simulink model "Slding control"  (R2020b)
settings: Solver=VariableStepAuto  StartTime=0.0  StopTime=50.0  RelTol=1e-3
values from neighbouring files (symbols this model uses):
  A = [-0.0239 -0.0494 0 -32.2 ... (first row only)    [P46091204.m]    (also in Sliding control.m)
  B = [0 ... (first row only)    [P46091204.m]    (also in Sliding control.m = [0 5.05*10^(-5))
  C = eye(4)    [P46091204.m]    (also in Sliding control.m = [K,eye(2)]*T)
  D = [0]    [P46091204.m]    (also in Sliding control.m = -C*A)
settings Model: Creator=ab458  LastModifiedBy=chengying
settings SolverCC: ZeroCrossAlgorithm=Adaptive
settings DebuggingCC: IgnoredZcDiagnostic=none
settings SFSimCC: CustomCodeUndefinedFunction=UseInterfaceOnly

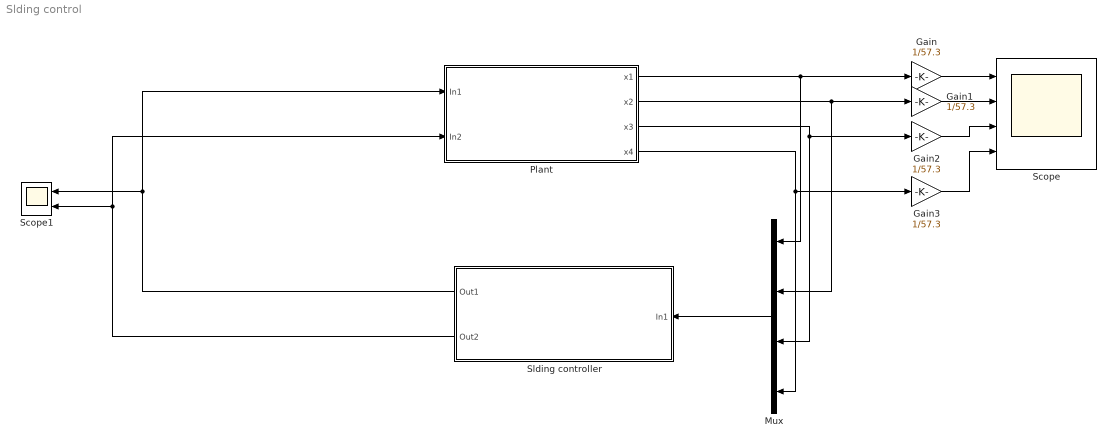
== system Slding control ==
  Gain{,1..3} (4 alike) : Gain  Gain=1/57.3
  Mux : Mux
  Plant : Subsystem
  Scope : Scope  NumInputPorts=4
  Scope1 : Scope  NumInputPorts=2
  Slding controller : Subsystem
  wires:
  Plant/1(x1) -> Mux/1, Gain/1
  Plant/2(x2) -> Mux/2, Gain1/1
  Plant/3(x3) -> Gain2/1, Mux/3
  Plant/4(x4) -> Gain3/1, Mux/4
  Slding controller/1(Out1) -> Plant/1(In1), Scope1/1
  Slding controller/2(Out2) -> Plant/2(In2), Scope1/2
  Mux/1 -> Slding controller/1(In1)
  Gain/1 -> Scope/1
  Gain1/1 -> Scope/2
  Gain2/1 -> Scope/3
  Gain3/1 -> Scope/4

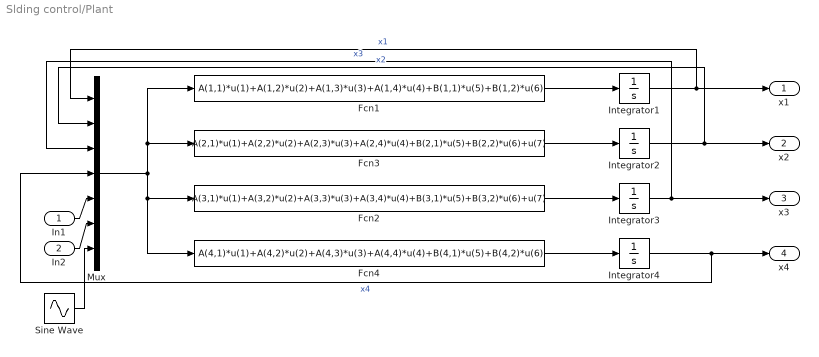
== system Slding control/Plant ==
  In1 : Inport
  In2 : Inport  Port=2
  Fcn1 : Fcn  Expr=A(1,1)*u(1)+A(1,2)*u(2)+A(1,3)*u(3)+A(1,4)*u(4)+B(1,1)*u(5)+B(1,2)*u(6)
  Fcn2 : Fcn  Expr=A(3,1)*u(1)+A(3,2)*u(2)+A(3,3)*u(3)+A(3,4)*u(4)+B(3,1)*u(5)+B(3,2)*u(6)+u(7)
  Fcn3 : Fcn  Expr=A(2,1)*u(1)+A(2,2)*u(2)+A(2,3)*u(3)+A(2,4)*u(4)+B(2,1)*u(5)+B(2,2)*u(6)+u(7)
  Fcn4 : Fcn  Expr=A(4,1)*u(1)+A(4,2)*u(2)+A(4,3)*u(3)+A(4,4)*u(4)+B(4,1)*u(5)+B(4,2)*u(6)
  Integrator1 : Integrator  InitialCondition=1
  Integrator2 : Integrator
  Integrator3 : Integrator  InitialCondition=1
  Integrator4 : Integrator
  Mux : Mux  Inputs=7
  Sine Wave : Sin  Amplitude=0.4  SampleTime=0
  x1 : Outport  VectorParamsAs1DForOutWhenUnconnected=off
  x2 : Outport  Port=2  VectorParamsAs1DForOutWhenUnconnected=off
  x3 : Outport  Port=3  VectorParamsAs1DForOutWhenUnconnected=off
  x4 : Outport  Port=4  VectorParamsAs1DForOutWhenUnconnected=off
  wires:
  Mux/1 -> Fcn3/1, Fcn1/1, Fcn4/1, Fcn2/1
  In2/1 -> Mux/6
  In1/1 -> Mux/5
  Fcn2/1 -> Integrator3/1
  Integrator1/1 -> x1/1, Mux/1  "x1"
  Integrator2/1 -> x2/1, Mux/2  "x2"
  Integrator4/1 -> x4/1, Mux/4  "x4"
  Fcn1/1 -> Integrator1/1
  Fcn4/1 -> Integrator4/1
  Integrator3/1 -> x3/1, Mux/3  "x3"
  Fcn3/1 -> Integrator2/1
  Sine Wave/1 -> Mux/7

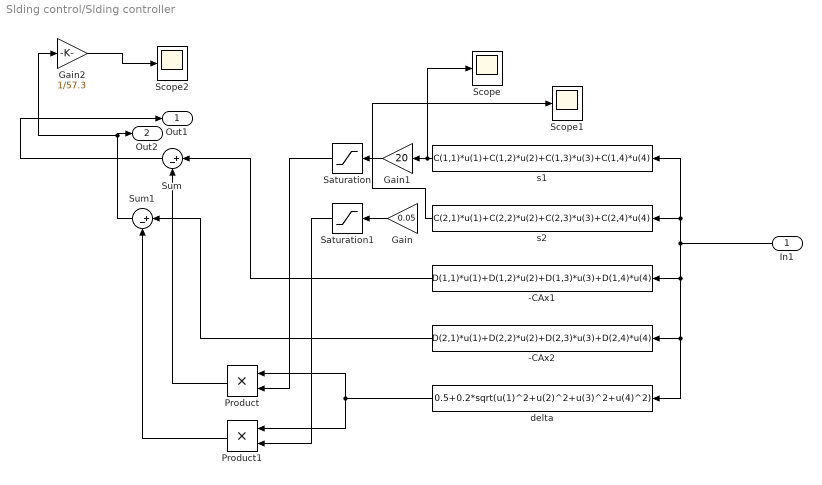
== system Slding control/Slding controller ==
  In1 : Inport
  -CAx1 : Fcn  Expr=D(1,1)*u(1)+D(1,2)*u(2)+D(1,3)*u(3)+D(1,4)*u(4)
  -CAx2 : Fcn  Expr=D(2,1)*u(1)+D(2,2)*u(2)+D(2,3)*u(3)+D(2,4)*u(4)
  Gain : Gain  Gain=0.05
  Gain1 : Gain  Gain=20
  Gain2 : Gain  Gain=1/57.3
  Product : Product
  Product1 : Product
  Saturation : Saturate
  Saturation1 : Saturate
  Scope : Scope
  Scope1 : Scope
  Scope2 : Scope
  Sum : Sum  Inputs=|+-
  Sum1 : Sum  Inputs=|+-
  delta : Fcn  Expr=0.5+0.2*sqrt(u(1)^2+u(2)^2+u(3)^2+u(4)^2)
  s1 : Fcn  Expr=C(1,1)*u(1)+C(1,2)*u(2)+C(1,3)*u(3)+C(1,4)*u(4)
  s2 : Fcn  Expr=C(2,1)*u(1)+C(2,2)*u(2)+C(2,3)*u(3)+C(2,4)*u(4)
  Out1 : Outport
  Out2 : Outport  Port=2
  wires:
  In1/1 -> delta/1, -CAx2/1, -CAx1/1, s2/1, s1/1
  s1/1 -> Scope/1, Gain1/1
  delta/1 -> Product1/1, Product/1
  Sum1/1 -> Gain2/1, Out2/1
  Product/1 -> Sum/2
  Product1/1 -> Sum1/2
  Saturation/1 -> Product/2
  Saturation1/1 -> Product1/2
  -CAx2/1 -> Sum1/1
  -CAx1/1 -> Sum/1
  Gain/1 -> Saturation1/1
  Gain1/1 -> Saturation/1
  Sum/1 -> Out1/1
  s2/1 -> Scope1/1
  Gain2/1 -> Scope2/1
